simulink model "Miniprojekt_Statespace"  (R2017b)
settings: Solver=VariableStepAuto  StartTime=0.0  StopTime=10000.0  RelTol=1e-3
values from neighbouring files (symbols this model uses):
  A = [ -(Cp*ro*fp+K1+Kw)/Cvw, K1/Cvw; K1/Cvp,-(K1+Kp)/Cvp]    [MP_Statespace.m]
  B = [ Cp*ro*fp/Cvw, Kw/Cvw; 0, Kp/Cvp ]    [MP_Statespace.m]
  C = [1,0;0,1]    [MP_Statespace.m]
  D = [0,0;0,0]    [MP_Statespace.m]
  dTz = 0    [MP_Statespace.m]
  dTzew = 2    [MP_Statespace.m]
  step_time = 1000    [MP_Statespace.m]
  Tz0 = Tz+3    (= 38)    [MP_Statespace.m]
  Tzew0 = Tzew+5    (= -2)    [MP_Statespace.m]
  X0 = [Twew0; Tp0]    [MP_Statespace.m]
settings Model: Creator=Piotr  LastModifiedBy=Piotr

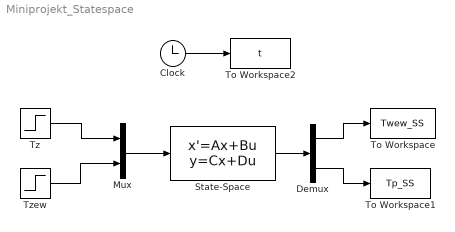
== system Miniprojekt_Statespace ==
  Clock : Clock
  Demux : Demux  Outputs=2
  Mux : Mux  Inputs=2
  State-Space : StateSpace  A=A  B=B  C=C  D=D  InitialCondition=X0
  To Workspace : ToWorkspace  VariableName=Twew_SS  SampleTime=-1
  To Workspace1 : ToWorkspace  VariableName=Tp_SS  SampleTime=-1
  To Workspace2 : ToWorkspace  VariableName=t  SampleTime=-1
  Tz : Step  Time=step_time  Before=Tz0  After=Tz0 + dTz  SampleTime=0
  "Tzew " : Step  Time=step_time  Before=Tzew0  After=Tzew0 + dTzew  SampleTime=0
  wires:
  Mux/1 -> State-Space/1
  State-Space/1 -> Demux/1
  "Tzew "/1 -> Mux/2
  Tz/1 -> Mux/1
  Demux/2 -> To Workspace1/1
  Demux/1 -> To Workspace/1
  Clock/1 -> To Workspace2/1
